simulink model "ANFIS_SIR_China_R2018b 2"  (R2018b)
settings: Solver=VariableStepAuto  StartTime=0.0  StopTime=90  RelTol=1e-3
undefined symbols (not defined in the file): beta
libraries: fuzblock x2, simulink x1
settings Model: Creator=ismae  LastModifiedBy=ismae
settings DataIOCC: ReturnWorkspaceOutputs=on

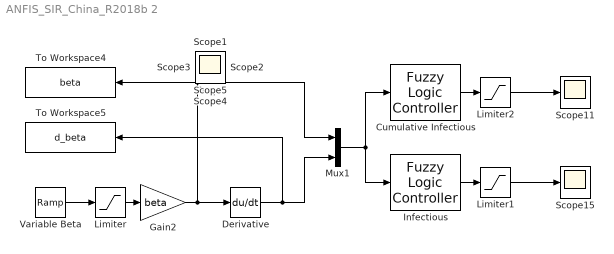
== system ANFIS_SIR_China_R2018b 2 ==
  Cumulative Infectious : fuzblock/Fuzzy Logic  Controller  FIS='FIS_C.fis'  OutputSampleNumber=101  DataType=double  FuzzifiedInputs=off  RuleFiringStrengths=off  RuleOutputs=off  AggregatedOutputs=off  SimulateUsing=Interpreted execution  OutOfRangeInputValueMessage=warning  NoRuleFiredMessage=warning  EmptyOutputFuzzySetMessage=warning
  Derivative : Derivative
  Gain2 : Gain  Gain=beta
  Infectious : fuzblock/Fuzzy Logic  Controller  FIS='FIS_I.fis'  OutputSampleNumber=101  DataType=double  FuzzifiedInputs=off  RuleFiringStrengths=off  RuleOutputs=off  AggregatedOutputs=off  SimulateUsing=Interpreted execution  OutOfRangeInputValueMessage=warning  NoRuleFiredMessage=warning  EmptyOutputFuzzySetMessage=warning
  Limiter : Saturate  UpperLimit=Inf  LowerLimit=0.3
  Limiter1 : Saturate  UpperLimit=Inf  LowerLimit=0  LinearizeAsGain=off  ZeroCross=off
  Limiter2 : Saturate  UpperLimit=Inf  LowerLimit=0  LinearizeAsGain=off  ZeroCross=off
  Mux1 : Mux  Inputs=2
  Scope{,1..5,11,15} (8 alike) : Scope
  To Workspace4 : ToWorkspace  VariableName=beta  SampleTime=1
      settings: Save2DSignal=2-D array (concatenate along first dimension)
  To Workspace5 : ToWorkspace  VariableName=d_beta  SampleTime=1
      settings: Save2DSignal=2-D array (concatenate along first dimension)
  Variable Beta : simulink/Sources/Ramp  slope=-0.00268  start=0  InitialOutput=0.7  VectorParams1D=off
  wires:
  Variable Beta/1 -> Limiter/1
  Limiter/1 -> Gain2/1
  Mux1/1 -> Cumulative Infectious/1, Infectious/1
  Cumulative Infectious/1 -> Limiter2/1
  Infectious/1 -> Limiter1/1
  Gain2/1 -> Derivative/1, Mux1/1, To Workspace4/1
  Limiter1/1 -> Scope15/1
  Limiter2/1 -> Scope11/1
  Derivative/1 -> Mux1/2, To Workspace5/1
